simulink model "cnn_closed_loop_model"  (R2023b)
settings: Solver=FixedStepAuto  StartTime=0.0  StopTime=149.8332  FixedStep=1/15000  RelTol=1e-3
InitFcn:
  | saveFolder = "Image Training Data Spectrogram";
  | load("Image Training Data Spectrogram\dataset.mat");
  | load("Controllers\controller_base.mat");
  | load("Controllers\notch_base.mat");
  | load("Image Training Data Spectrogram\normalization_stats.mat");
  | load("Models\ResNet18_Spectrogram_trained.mat");
  | simTime = 6.6667e-05 * (length(results)-1);
values from neighbouring files (symbols this model uses):
  results = struct('image', {}, 'target', {})    [Scalogram.m]    (also in Spectrogram.m; predict.m = table('Size', [numel(fileList), 4],      'VariableTypes', {')
undefined symbols (not defined in the file or in its folder): targetMean, targetStd
libraries: cstblocks x2, deeplib x1
settings Model: Creator=MUSTAFAUGUR  LastModifiedBy=MUSTAFAUGUR
settings DebuggingCC: ParameterPrecisionLossMsg=none

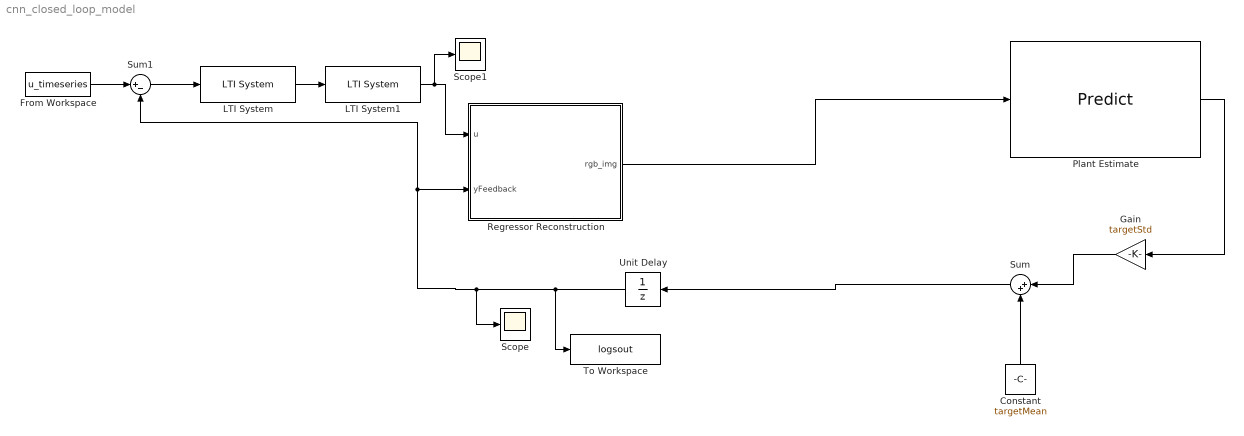
== system cnn_closed_loop_model ==
  Constant : Constant  Value=targetMean
  From Workspace : FromWorkspace  VariableName=u_timeseries
  Gain : Gain  Gain=targetStd
  LTI System : cstblocks/LTI System  sys=C_optd  IC=[]  PadeOrder=0
  LTI System1 : cstblocks/LTI System  sys=notchD  IC=[]  PadeOrder=0
  Plant Estimate : deeplib/Predict  Network=Network from MAT-file  NetworkFunction=squeezenet  NetworkFilePath=C:\Users\MUSTAFAUGUR\Desktop\ArdaGencer\Models\ResNet18_Spectrogram_trained.mat  MiniBatchSize=64  InputDataFormats={'',''}  Predictions=on  Activations={}  ForceInterpretedSim=off  EnableDLNetwork=on
  Regressor Reconstruction : MATLAB Function  TreatAsAtomicUnit=on
  Scope : Scope
  Scope1 : Scope
  Sum : Sum  Inputs=|++
  Sum1 : Sum  Inputs=|+-
  To Workspace : ToWorkspace  VariableName=logsout  SaveFormat=Timeseries  SampleTime=-1
  Unit Delay : UnitDelay  SampleTime=-1  HasFrameUpgradeWarning=on
  wires:
  Regressor Reconstruction/1(rgb_img) -> Plant Estimate/1
  LTI System/1 -> LTI System1/1
  LTI System1/1 -> Scope1/1, Regressor Reconstruction/1(u)
  Unit Delay/1 -> To Workspace/1, Scope/1, Regressor Reconstruction/2(yFeedback), Sum1/2
  Plant Estimate/1 -> Gain/1
  From Workspace/1 -> Sum1/1
  Sum1/1 -> LTI System/1
  Gain/1 -> Sum/1
  Constant/1 -> Sum/2
  Sum/1 -> Unit Delay/1

== matlab function cnn_closed_loop_model/Regressor Reconstruction ==
  data: u input; rgb_img output; yFeedback input
function rgb_img = spectrogramImageBlock(u, yFeedback)
coder.extrinsic('spectrogram','gray2ind','ind2rgb','loadStats','hamming','parula');

persistent uBuffer yBuffer muU sigmaU muYimg sigmaYimg initialized
persistent hammingWin callCounter cachedImg cmap

windowSize = 200;
sttWindowSamples = 64;
sttOverlapSamples = round(0.9*sttWindowSamples);
sttNfft = 128;
Fs = 15000;
nStd = 3;
statsPath = 'Image Training Data Spectrogram/normalization_stats.mat';
hopSamples = sttWindowSamples - sttOverlapSamples;

numRows = floor(sttNfft/2) + 1;
numCols = floor((windowSize - sttOverlapSamples) / (sttWindowSamples - sttOverlapSamples));

muU = 0; sigmaU = 1; muYimg = 0; sigmaYimg = 1;

if isempty(initialized)
    uBuffer = zeros(windowSize,1);
    yBuffer = zeros(windowSize,1);
    hammingWin = hamming(sttWindowSamples);
    cmap = parula(256);
    [muU, sigmaU, muYimg, sigmaYimg] = loadStats(statsPath);
    callCounter = 0;
    cachedImg = zeros(2*numRows, numCols, 3);
    initialized = true;
end

uBuffer = [uBuffer(2:end); u];
yBuffer = [yBuffer(2:end); yFeedback];
callCounter = callCounter + 1;

if callCounter >= hopSamples
    callCounter = 0;

    s_u = complex(zeros(numRows, numCols));
    s_y = complex(zeros(numRows, numCols));
    s_u = spectrogram(uBuffer, hammingWin, sttOverlapSamples, sttNfft, Fs);
    s_y = spectrogram(yBuffer, hammingWin, sttOverlapSamples, sttNfft, Fs);
    s_mag_u = 10*log10(abs(s_u)+eps);
    s_mag_y = 10*log10(abs(s_y)+eps);

    z_u = max(-nStd, min(nStd, (s_mag_u-muU)/sigmaU));
    z_y = max(-nStd, min(nStd, (s_mag_y-muYimg)/sigmaYimg));
    u_norm = (z_u+nStd)/(2*nStd);
    y_norm = (z_y+nStd)/(2*nStd);
    combined = [u_norm; y_norm];

    ind_img = zeros(2*numRows, numCols, 'uint8');
    ind_img = gray2ind(combined, 256);
    cachedImg = ind2rgb(ind_img, cmap);
end

rgb_img = cachedImg;
